simulink model "BLDCBlockTest"  (R2020a)
settings: Solver=VariableStepAuto  StartTime=0.0  StopTime=1.0  RelTol=1e-3
libraries: fl_lib x33, nesl_utility x9, eeTransforms x3, ee_lib x2, mcbcontrolslib x1, mcbpositiondecoderlib x1
settings Model: Creator=enzoe  LastModifiedBy=enzoe

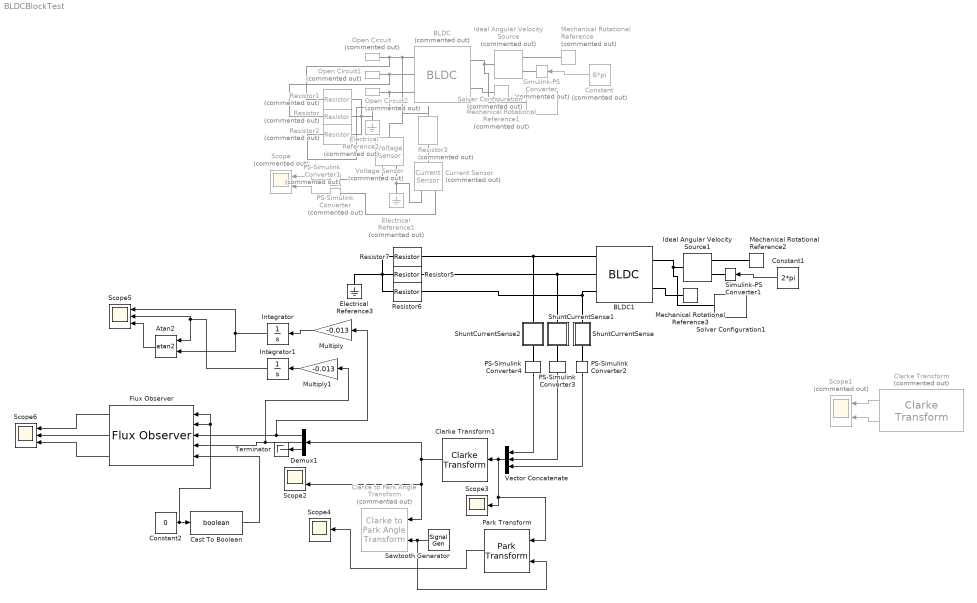
== system BLDCBlockTest ==
  Atan2 : Trigonometry  Operator=atan2
  BLDC : ee_lib/Electromechanical/Permanent Magnet/BLDC  Commented=on  winding_type=ee.enum.statorconnection.delta  rotor_param=2  pm_flux_linkage=1 Wb  theta_constant=pi/12 rad  emf_max=9.6 V  DphiDtheta_tab=[0, -.1528, -.1528, .1528, .1528, 0] Wb/rad  back_emf_tab=[0, -9.6, -9.6, 9.6, 9.6, 0] V  rotor_angle_tab=[0, 7.5, 22.5, 37.5, 52.5, 60] deg  w_meas=600 rpm  nPolePairs=6  stator_param=ee.enum.statorparam.LdLqL0  machine_param=ee.enum.dqparameterization.constant  Ld=0.00022 H  Lq=0.00022 H  idVec=[-200, 0, 200] A  iqVec=[-200, 0, 200] A  LdMatrix=0.00022 * ones(3, 3) H  LqMatrix=0.00022 * ones(3, 3) H  L0=0.00016 H  Ls=0.0002 H  Lm=0 H  Ms=0.00002 H  Rs=0.013 Ohm  zero_sequence=ee.enum.park.zerosequence.include  J=0.01 kg*m^2  lam=0 N*m/(rad/s)  axes_param=2  i_d_specify=off  i_d_priority=None  i_d=0 A  i_d_nominal_specify=off  i_d_nominal_unit=A  i_d_nominal_value=1  i_q_specify=off  i_q_priority=None  i_q=0 A  i_q_nominal_specify=off  i_q_nominal_unit=A  i_q_nominal_value=1  torque_specify=off  torque_priority=None  torque=0 N*m  torque_nominal_specify=off  torque_nominal_unit=N*m  torque_nominal_value=1  angular_velocity_specify=off  angular_velocity_priority=High  angular_velocity=0 rpm  angular_velocity_nominal_specify=off  angular_velocity_nominal_unit=rpm  angular_velocity_nominal_value=1  angular_position_specify=off  angular_position_priority=High  angular_position=0 deg  angular_position_nominal_specify=off  angular_position_nominal_unit=deg  angular_position_nominal_value=1  loss_param=ee.enum.ironloss.none  losses_oc=[0, 0, 0] W  losses_sc=[0, 0, 0] W  f_losses=60 Hz  Isc_losses=95 A  Tmeas=298.15 K  alpha=3.93e-3 1/K  alpha_flux=-0.001 1/K  stator_thermal_mass=100 J/K  rotor_thermal_mass=200 J/K  Rm_percent_rotor=90  Rd_percent_rotor=30  temperatureA_specify=off  temperatureA_priority=High  temperatureA=25 degC  temperatureA_nominal_specify=off  temperatureA_nominal_unit=degC  temperatureA_nominal_value=1  temperatureB_specify=off  temperatureB_priority=High  temperatureB=25 degC  temperatureB_nominal_specify=off  temperatureB_nominal_unit=degC  temperatureB_nominal_value=1  temperatureC_specify=off  temperatureC_priority=High  temperatureC=25 degC  temperatureC_nominal_specify=off  temperatureC_nominal_unit=degC  temperatureC_nominal_value=1  temperatureR_specify=off  temperatureR_priority=High  temperatureR=25 degC  temperatureR_nominal_specify=off  temperatureR_nominal_unit=degC  temperatureR_nominal_value=1
      settings: SourceProductBaseCode=PS  InternalSimscapePortConfiguration="{\"Bottom\":[],\"Left\":[{\"id\":\"a\",\"label\":\"a\",\"type\":\"foundation.electrical.electrical\"},{\"id\":\"b\",\"label\":\"b\",\"type\":\"foundation.electrical.electrical\"},{\"id\":\"c\",\"label\":\"c\",\"type\":\"foundation.electrical.electrical\"}],\"Right\":[{\"id\":\"R\",\"label\":\"R\",\"type\":\"foundation.mechanical.rotational.rotational\"},{\"id\":\"C\",\"label\":\"C\",\"type\":\"foundation.mechanical.rotational.rotational\"}],\"Top\":[]}"
  BLDC1 : ee_lib/Electromechanical/Permanent Magnet/BLDC  winding_type=ee.enum.statorconnection.delta  rotor_param=2  pm_flux_linkage=1 Wb  theta_constant=pi/2 rad  emf_max=9.6 V  DphiDtheta_tab=[0, -.1528, -.1528, .1528, .1528, 0] Wb/rad  back_emf_tab=[0, -9.6, -9.6, 9.6, 9.6, 0] V  rotor_angle_tab=[0, 7.5, 22.5, 37.5, 52.5, 60] deg  w_meas=600 rpm  nPolePairs=1  stator_param=ee.enum.statorparam.LdLqL0  machine_param=ee.enum.dqparameterization.constant  Ld=0.00022 H  Lq=0.00022 H  idVec=[-200, 0, 200] A  iqVec=[-200, 0, 200] A  LdMatrix=0.00022 * ones(3, 3) H  LqMatrix=0.00022 * ones(3, 3) H  L0=0.00016 H  Ls=0.0002 H  Lm=0 H  Ms=0.00002 H  Rs=0.013 Ohm  zero_sequence=ee.enum.park.zerosequence.include  J=0.01 kg*m^2  lam=0 N*m/(rad/s)  axes_param=2  i_d_specify=off  i_d_priority=None  i_d=0 A  i_d_nominal_specify=off  i_d_nominal_unit=A  i_d_nominal_value=1  i_q_specify=off  i_q_priority=None  i_q=0 A  i_q_nominal_specify=off  i_q_nominal_unit=A  i_q_nominal_value=1  torque_specify=off  torque_priority=None  torque=0 N*m  torque_nominal_specify=off  torque_nominal_unit=N*m  torque_nominal_value=1  angular_velocity_specify=off  angular_velocity_priority=High  angular_velocity=0 rpm  angular_velocity_nominal_specify=off  angular_velocity_nominal_unit=rpm  angular_velocity_nominal_value=1  angular_position_specify=off  angular_position_priority=High  angular_position=0 deg  angular_position_nominal_specify=off  angular_position_nominal_unit=deg  angular_position_nominal_value=1  loss_param=ee.enum.ironloss.none  losses_oc=[0, 0, 0] W  losses_sc=[0, 0, 0] W  f_losses=60 Hz  Isc_losses=95 A  Tmeas=298.15 K  alpha=3.93e-3 1/K  alpha_flux=-0.001 1/K  stator_thermal_mass=100 J/K  rotor_thermal_mass=200 J/K  Rm_percent_rotor=90  Rd_percent_rotor=30  temperatureA_specify=off  temperatureA_priority=High  temperatureA=25 degC  temperatureA_nominal_specify=off  temperatureA_nominal_unit=degC  temperatureA_nominal_value=1  temperatureB_specify=off  temperatureB_priority=High  temperatureB=25 degC  temperatureB_nominal_specify=off  temperatureB_nominal_unit=degC  temperatureB_nominal_value=1  temperatureC_specify=off  temperatureC_priority=High  temperatureC=25 degC  temperatureC_nominal_specify=off  temperatureC_nominal_unit=degC  temperatureC_nominal_value=1  temperatureR_specify=off  temperatureR_priority=High  temperatureR=25 degC  temperatureR_nominal_specify=off  temperatureR_nominal_unit=degC  temperatureR_nominal_value=1
      settings: SourceProductBaseCode=PS  InternalSimscapePortConfiguration="{\"Bottom\":[],\"Left\":[{\"id\":\"a\",\"label\":\"a\",\"type\":\"foundation.electrical.electrical\"},{\"id\":\"b\",\"label\":\"b\",\"type\":\"foundation.electrical.electrical\"},{\"id\":\"c\",\"label\":\"c\",\"type\":\"foundation.electrical.electrical\"}],\"Right\":[{\"id\":\"R\",\"label\":\"R\",\"type\":\"foundation.mechanical.rotational.rotational\"},{\"id\":\"C\",\"label\":\"C\",\"type\":\"foundation.mechanical.rotational.rotational\"}],\"Top\":[]}"
  Cast To Boolean : DataTypeConversion  OutDataTypeStr=boolean
  Clarke Transform : mcbcontrolslib/Clarke Transform  Commented=on  VariantControl=Variant2
  Clarke Transform1 : eeTransforms/Clarke Transform  PowerInvariant=on
      settings: SourceProductBaseCode=PS
  Clarke to Park Angle Transform : eeTransforms/Clarke to Park Angle Transform  Commented=on  AxisAlignment=D-axis
      settings: SourceProductBaseCode=PS
  Constant : Constant  Commented=on  Value=6*pi
  Constant1 : Constant  Value=2*pi
  Constant2 : Constant  Value=0
  Current Sensor : fl_lib/Electrical/Electrical Sensors/Current Sensor  Commented=on
  Demux1 : Demux  Outputs=3
  Electrical Reference1 : fl_lib/Electrical/Electrical Elements/Electrical Reference  Commented=on
  Electrical Reference2 : fl_lib/Electrical/Electrical Elements/Electrical Reference  Commented=on
  Electrical Reference3 : fl_lib/Electrical/Electrical Elements/Electrical Reference
  Flux Observer : mcbpositiondecoderlib/Flux Observer  BlockInputUnit=SI unit  PerUnitVoltage=13.86  PerUnitCurrent=19.3  PositionSelect=on  FluxSelect=on  TorqueSelect=on  PolePairs=1  StatorResistance=0.013  BlockSampleTime=50e-6  PositionUnit=Radians  PositionDatatype=single  FluxUnit=Weber  PerUnitFlux=0.1  FluxDatatype=single  TorqueUnit=Nm  PerUnitTorque=100  TorqueDatatype=single
      settings: SourceProductBaseCode=MT
  Ideal Angular Velocity Source : fl_lib/Mechanical/Mechanical Sources/Ideal Angular Velocity Source  Commented=on
  Ideal Angular Velocity Source1 : fl_lib/Mechanical/Mechanical Sources/Ideal Angular Velocity Source
  Integrator : Integrator
  Integrator1 : Integrator
  Mechanical Rotational Reference : fl_lib/Mechanical/Rotational Elements/Mechanical Rotational Reference  Commented=on
  Mechanical Rotational Reference1 : fl_lib/Mechanical/Rotational Elements/Mechanical Rotational Reference  Commented=on
  Mechanical Rotational Reference2 : fl_lib/Mechanical/Rotational Elements/Mechanical Rotational Reference
  Mechanical Rotational Reference3 : fl_lib/Mechanical/Rotational Elements/Mechanical Rotational Reference
  Multiply : Gain  Gain=-0.013
  Multiply1 : Gain  Gain=-0.013
  Open Circuit : fl_lib/Electrical/Electrical Elements/Open Circuit  Commented=on  v_specify=off  v_priority=None  v=0 V  v_nominal_specify=off  v_nominal_unit=V  v_nominal_value=1
      settings: SourceProductBaseCode=SS
  Open Circuit1 : fl_lib/Electrical/Electrical Elements/Open Circuit  Commented=on  v_specify=off  v_priority=None  v=0 V  v_nominal_specify=off  v_nominal_unit=V  v_nominal_value=1
      settings: SourceProductBaseCode=SS
  Open Circuit2 : fl_lib/Electrical/Electrical Elements/Open Circuit  Commented=on  v_specify=off  v_priority=None  v=0 V  v_nominal_specify=off  v_nominal_unit=V  v_nominal_value=1
      settings: SourceProductBaseCode=SS
  PS-Simulink Converter : nesl_utility/PS-Simulink Converter  Commented=on  PhysicalDomain=network_engine_domain  SubClassName=ps_output  LeftPortType=input  RightPortType=output  PseudoPeriodic=off  Frequencies=[]  Unit=inherit  AffineConversion=off
  PS-Simulink Converter1 : nesl_utility/PS-Simulink Converter  Commented=on  PhysicalDomain=network_engine_domain  SubClassName=ps_output  LeftPortType=input  RightPortType=output  PseudoPeriodic=off  Frequencies=[]  Unit=inherit  AffineConversion=off
  PS-Simulink Converter2 : nesl_utility/PS-Simulink Converter  PhysicalDomain=network_engine_domain  SubClassName=ps_output  LeftPortType=input  RightPortType=output  PseudoPeriodic=off  Frequencies=[]  Unit=inherit  AffineConversion=off
  PS-Simulink Converter3 : nesl_utility/PS-Simulink Converter  PhysicalDomain=network_engine_domain  SubClassName=ps_output  LeftPortType=input  RightPortType=output  PseudoPeriodic=off  Frequencies=[]  Unit=inherit  AffineConversion=off
  PS-Simulink Converter4 : nesl_utility/PS-Simulink Converter  PhysicalDomain=network_engine_domain  SubClassName=ps_output  LeftPortType=input  RightPortType=output  PseudoPeriodic=off  Frequencies=[]  Unit=inherit  AffineConversion=off
  Park Transform : eeTransforms/Park Transform  AxisAlignment=D-axis  PowerInvariant=off
  Resistor : fl_lib/Electrical/Electrical Elements/Resistor  Commented=on  R=1000000 Ohm  i_specify=off  i_priority=None  i=0 A  i_nominal_specify=off  i_nominal_unit=A  i_nominal_value=1  v_specify=off  v_priority=None  v=0 V  v_nominal_specify=off  v_nominal_unit=V  v_nominal_value=1
  Resistor1 : fl_lib/Electrical/Electrical Elements/Resistor  Commented=on  R=1000000 Ohm  i_specify=off  i_priority=None  i=0 A  i_nominal_specify=off  i_nominal_unit=A  i_nominal_value=1  v_specify=off  v_priority=None  v=0 V  v_nominal_specify=off  v_nominal_unit=V  v_nominal_value=1
  Resistor2 : fl_lib/Electrical/Electrical Elements/Resistor  Commented=on  R=1000000 Ohm  i_specify=off  i_priority=None  i=0 A  i_nominal_specify=off  i_nominal_unit=A  i_nominal_value=1  v_specify=off  v_priority=None  v=0 V  v_nominal_specify=off  v_nominal_unit=V  v_nominal_value=1
  Resistor3 : fl_lib/Electrical/Electrical Elements/Resistor  Commented=on  R=10 Ohm  i_specify=off  i_priority=None  i=0 A  i_nominal_specify=off  i_nominal_unit=A  i_nominal_value=1  v_specify=off  v_priority=None  v=0 V  v_nominal_specify=off  v_nominal_unit=V  v_nominal_value=1
  Resistor5 : fl_lib/Electrical/Electrical Elements/Resistor  R=100 Ohm  i_specify=off  i_priority=None  i=0 A  i_nominal_specify=off  i_nominal_unit=A  i_nominal_value=1  v_specify=off  v_priority=None  v=0 V  v_nominal_specify=off  v_nominal_unit=V  v_nominal_value=1
  Resistor6 : fl_lib/Electrical/Electrical Elements/Resistor  R=100 Ohm  i_specify=off  i_priority=None  i=0 A  i_nominal_specify=off  i_nominal_unit=A  i_nominal_value=1  v_specify=off  v_priority=None  v=0 V  v_nominal_specify=off  v_nominal_unit=V  v_nominal_value=1
  Resistor7 : fl_lib/Electrical/Electrical Elements/Resistor  R=100 Ohm  i_specify=off  i_priority=None  i=0 A  i_nominal_specify=off  i_nominal_unit=A  i_nominal_value=1  v_specify=off  v_priority=None  v=0 V  v_nominal_specify=off  v_nominal_unit=V  v_nominal_value=1
  Sawtooth Generator : SignalGenerator  WaveForm=sawtooth  Amplitude=360  Frequency=2  Units=rad/sec
  Scope : Scope  Commented=on  NumInputPorts=2
  Scope1 : Scope  Commented=on  NumInputPorts=2
  Scope2 : Scope  NumInputPorts=2
  Scope3 : Scope
  Scope4 : Scope
  Scope5 : Scope  NumInputPorts=3
  Scope6 : Scope  NumInputPorts=3
  ShuntCurrentSense : Subsystem
  ShuntCurrentSense1 : Subsystem
  ShuntCurrentSense2 : Subsystem
  Simulink-PS Converter : nesl_utility/Simulink-PS Converter  Commented=on  PhysicalDomain=network_engine_domain  SubClassName=ps_input  LeftPortType=input  RightPortType=output  PseudoPeriodic=off  Frequencies=[]  NoiseDistribution=none  NoiseParameters=[]  Unit=1  AffineConversion=off  FilteringAndDerivatives=provide  SimscapeFilterOrder=1  InputFilterTimeConstant=0.001  UdotUserProvided=0
  Simulink-PS Converter1 : nesl_utility/Simulink-PS Converter  PhysicalDomain=network_engine_domain  SubClassName=ps_input  LeftPortType=input  RightPortType=output  PseudoPeriodic=off  Frequencies=[]  NoiseDistribution=none  NoiseParameters=[]  Unit=1  AffineConversion=off  FilteringAndDerivatives=provide  SimscapeFilterOrder=1  InputFilterTimeConstant=0.001  UdotUserProvided=0
  Solver Configuration : nesl_utility/Solver Configuration  Commented=on  PhysicalDomain=network_engine_domain  SubClassName=solver  LeftPortType=input  RightPortType=generic  Tones=[]  Harmonics=[]  SimulateNoise=off  Profile=off  UseLocalSampling=off  EnableSwitchedLinearOptims=on  FrequencyDomain=off  UseCCode=off  RelTol=0.001  AbsTol=1e-06  MinStep=1e-09  ToWorkspace=off  RevertToSquareIcSolve=off  NumHomotopyIterations=100  PhasorMode=off  PhasorModeNumHarmonics=1  DoDC=off  ResidualTolerance=1e-09  UseLocalSolver=on  LocalSolverChoice=NE_BACKWARD_EULER_ADVANCER  LocalSolverSampleTime=2e-6  DoFixedCost=on  MaxNonlinIter=3  MaxModeIter=2  LinearAlgebra=auto  EquationFormulation=NE_TIME_EF  DelaysMemoryBudget=1024  AutomaticFiltering=on  FilteringTimeConstant=0.001  PartitionStorageMethod=AS_NEEDED  PartitionMemoryBudget=1024  PartitionMethod=ROBUST
  Solver Configuration1 : nesl_utility/Solver Configuration  PhysicalDomain=network_engine_domain  SubClassName=solver  LeftPortType=input  RightPortType=generic  Tones=[]  Harmonics=[]  SimulateNoise=off  Profile=off  UseLocalSampling=off  EnableSwitchedLinearOptims=on  FrequencyDomain=off  UseCCode=off  RelTol=0.001  AbsTol=1e-06  MinStep=1e-09  ToWorkspace=off  RevertToSquareIcSolve=off  NumHomotopyIterations=100  PhasorMode=off  PhasorModeNumHarmonics=1  DoDC=off  ResidualTolerance=1e-09  UseLocalSolver=on  LocalSolverChoice=NE_BACKWARD_EULER_ADVANCER  LocalSolverSampleTime=2e-6  DoFixedCost=on  MaxNonlinIter=3  MaxModeIter=2  LinearAlgebra=auto  EquationFormulation=NE_TIME_EF  DelaysMemoryBudget=1024  AutomaticFiltering=on  FilteringTimeConstant=0.001  PartitionStorageMethod=AS_NEEDED  PartitionMemoryBudget=1024  PartitionMethod=ROBUST
  Terminator : Terminator
  Vector Concatenate : Concatenate  NumInputs=3
  Voltage Sensor : fl_lib/Electrical/Electrical Sensors/Voltage Sensor  Commented=on
  wires:
  Constant/1 -> Simulink-PS Converter/1
  PS-Simulink Converter/1 -> Scope/1
  PS-Simulink Converter1/1 -> Scope/2
  Constant1/1 -> Simulink-PS Converter1/1
  Clarke Transform/1 -> Scope1/1
  Clarke Transform/2 -> Scope1/2
  PS-Simulink Converter4/1 -> Vector Concatenate/1
  PS-Simulink Converter3/1 -> Vector Concatenate/2
  PS-Simulink Converter2/1 -> Vector Concatenate/3
  Vector Concatenate/1 -> Park Transform/1, Scope3/1, Clarke Transform1/1
  Clarke Transform1/1 -> Clarke to Park Angle Transform/1, Scope2/2, Demux1/1
  Sawtooth Generator/1 -> Park Transform/2, Clarke to Park Angle Transform/2
  Park Transform/1 -> Scope4/1
  Demux1/1 -> Multiply/1, Flux Observer/3
  Demux1/2 -> Multiply1/1, Flux Observer/4
  Constant2/1 -> Flux Observer/1, Flux Observer/2, Cast To Boolean/1
  Cast To Boolean/1 -> Flux Observer/5
  Flux Observer/1 -> Scope6/1
  Multiply/1 -> Integrator/1
  Demux1/3 -> Terminator/1
  Integrator/1 -> Scope5/1, Atan2/2
  Flux Observer/2 -> Scope6/2
  Flux Observer/3 -> Scope6/3
  Multiply1/1 -> Integrator1/1
  Integrator1/1 -> Atan2/1, Scope5/2
  Atan2/1 -> Scope5/3
  connections:
  Open Circuit/LConn1 -- Resistor3/LConn1 -- Voltage Sensor/LConn1 -- BLDC/LConn1 -- Resistor1/LConn1
  BLDC/LConn2 -- Resistor/LConn1 -- Open Circuit1/LConn1
  BLDC/LConn3 -- Resistor2/LConn1 -- Open Circuit2/LConn1
  Ideal Angular Velocity Source/LConn1 -- BLDC/RConn1 -- Solver Configuration/RConn1
  Mechanical Rotational Reference/LConn1 -- Ideal Angular Velocity Source/RConn2
  Simulink-PS Converter/RConn1 -- Ideal Angular Velocity Source/RConn1
  Voltage Sensor/RConn1 -- PS-Simulink Converter/LConn1
  Mechanical Rotational Reference1/LConn1 -- BLDC/RConn2
  Resistor1/RConn1 -- Electrical Reference2/LConn1 -- Resistor2/RConn1 -- Resistor/RConn1
  Current Sensor/RConn1 -- PS-Simulink Converter1/LConn1
  Current Sensor/RConn2 -- Voltage Sensor/RConn2 -- Electrical Reference1/LConn1
  Resistor3/RConn1 -- Current Sensor/LConn1
  Resistor6/LConn1 -- ShuntCurrentSense/LConn1 -- BLDC1/LConn3
  Resistor5/LConn1 -- ShuntCurrentSense1/LConn1 -- BLDC1/LConn2
  Ideal Angular Velocity Source1/LConn1 -- BLDC1/RConn1 -- Solver Configuration1/RConn1
  Mechanical Rotational Reference3/LConn1 -- BLDC1/RConn2
  Simulink-PS Converter1/RConn1 -- Ideal Angular Velocity Source1/RConn1
  Mechanical Rotational Reference2/LConn1 -- Ideal Angular Velocity Source1/RConn2
  Resistor5/RConn1 -- Electrical Reference3/LConn1 -- Resistor7/RConn1 -- Resistor6/RConn1
  Resistor7/LConn1 -- ShuntCurrentSense2/LConn1 -- BLDC1/LConn1
  PS-Simulink Converter2/LConn1 -- ShuntCurrentSense/RConn1
  PS-Simulink Converter3/LConn1 -- ShuntCurrentSense1/RConn1
  PS-Simulink Converter4/LConn1 -- ShuntCurrentSense2/RConn1

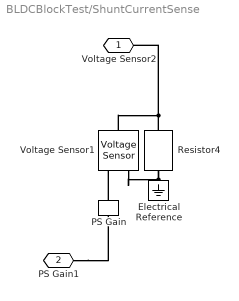
== system BLDCBlockTest/ShuntCurrentSense ==
  Electrical Reference : fl_lib/Electrical/Electrical Elements/Electrical Reference
  PS Gain : fl_lib/Physical Signals/Functions/PS Gain  gain=1
  Resistor4 : fl_lib/Electrical/Electrical Elements/Resistor  R=1 Ohm  i_specify=off  i_priority=None  i=0 A  i_nominal_specify=off  i_nominal_unit=A  i_nominal_value=1  v_specify=off  v_priority=None  v=0 V  v_nominal_specify=off  v_nominal_unit=V  v_nominal_value=1
  Voltage Sensor1 : fl_lib/Electrical/Electrical Sensors/Voltage Sensor
  Voltage Sensor2 : PMIOPort  Side=Left
  PS Gain1 : PMIOPort  Port=2  Side=Right
  connections:
  PS Gain1/RConn1 -- PS Gain/RConn1
  Electrical Reference/LConn1 -- Voltage Sensor1/RConn2 -- Resistor4/RConn1
  Resistor4/LConn1 -- Voltage Sensor2/RConn1 -- Voltage Sensor1/LConn1
  PS Gain/LConn1 -- Voltage Sensor1/RConn1

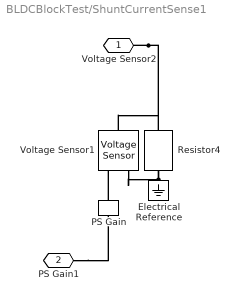
== system BLDCBlockTest/ShuntCurrentSense1 ==
  Electrical Reference : fl_lib/Electrical/Electrical Elements/Electrical Reference
  PS Gain : fl_lib/Physical Signals/Functions/PS Gain  gain=1
  Resistor4 : fl_lib/Electrical/Electrical Elements/Resistor  R=1 Ohm  i_specify=off  i_priority=None  i=0 A  i_nominal_specify=off  i_nominal_unit=A  i_nominal_value=1  v_specify=off  v_priority=None  v=0 V  v_nominal_specify=off  v_nominal_unit=V  v_nominal_value=1
  Voltage Sensor1 : fl_lib/Electrical/Electrical Sensors/Voltage Sensor
  Voltage Sensor2 : PMIOPort  Side=Left
  PS Gain1 : PMIOPort  Port=2  Side=Right
  connections:
  PS Gain/LConn1 -- Voltage Sensor1/RConn1
  Voltage Sensor2/RConn1 -- Resistor4/LConn1 -- Voltage Sensor1/LConn1
  Voltage Sensor1/RConn2 -- Resistor4/RConn1 -- Electrical Reference/LConn1
  PS Gain1/RConn1 -- PS Gain/RConn1

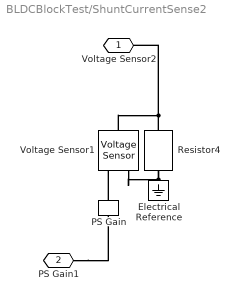
== system BLDCBlockTest/ShuntCurrentSense2 ==
  Electrical Reference : fl_lib/Electrical/Electrical Elements/Electrical Reference
  PS Gain : fl_lib/Physical Signals/Functions/PS Gain  gain=1
  Resistor4 : fl_lib/Electrical/Electrical Elements/Resistor  R=1 Ohm  i_specify=off  i_priority=None  i=0 A  i_nominal_specify=off  i_nominal_unit=A  i_nominal_value=1  v_specify=off  v_priority=None  v=0 V  v_nominal_specify=off  v_nominal_unit=V  v_nominal_value=1
  Voltage Sensor1 : fl_lib/Electrical/Electrical Sensors/Voltage Sensor
  Voltage Sensor2 : PMIOPort  Side=Left
  PS Gain1 : PMIOPort  Port=2  Side=Right
  connections:
  PS Gain1/RConn1 -- PS Gain/RConn1
  Electrical Reference/LConn1 -- Resistor4/RConn1 -- Voltage Sensor1/RConn2
  Voltage Sensor1/LConn1 -- Resistor4/LConn1 -- Voltage Sensor2/RConn1
  PS Gain/LConn1 -- Voltage Sensor1/RConn1
